simulink model "buses_snt"  (R2025b)
settings: Solver=ode45  StartTime=0.0  StopTime=10.0  RelTol=1e-3  EnableMultiTasking=on
undefined symbols (not defined in the file or in its folder): Rg, Ts
libraries: fl_lib x12, nesl_utility x12, ee_lib x6, eeRmsMeasurement x3
settings Model: Creator=gdudgeon  LastModifiedBy=gdudgeon
settings SolverCC: AlgebraicLoopSolver=TrustRegion
settings DataIOCC: LimitDataPoints=on  SaveFormat=Array  ReturnWorkspaceOutputs=off
settings OptimizationCC: ExpressionDepthLimit=2147483647.0  LifeSpan=inf
settings DebuggingCC: UnderspecifiedInitializationDetection=Classic  MergeDetectMultiDrivingBlocksExec=none  SolverPrmCheckMsg=warning  UnconnectedInputMsg=warning  UnconnectedOutputMsg=warning  UnconnectedLineMsg=warning  StateNameClashWarn=warning  SFUnexpectedBacktrackingDiag=warning  SFNoUnconditionalDefaultTransitionDiag=warning  SFExecutionAtInitializationDiag=none  ArithmeticOperatorsInVariantConditions=warning
settings HardwareCC: ProdBitPerPointer=32.0  ProdBitPerSizeT=32.0  ProdBitPerPtrDiffT=32.0  ProdLargestAtomicFloat=None  ProdIntDivRoundTo=Undefined  ProdEndianess=Unspecified  ProdWordSize=32.0  ProdHWDeviceType=32-bit Generic
settings ModelReferenceCC: EnableRefExpFcnMdlSchedulingChecks=on  PropagateSignalLabelsOutOfModel=off
settings SFSimCC: SimUseLocalCustomCode=off  CustomCodeUndefinedFunction=UseInterfaceOnly
settings RTWCC: RTWUseLocalCustomCode=off  GPUComputeCapability=3.5
settings CodeAppCC: StateflowObjectComments=on
settings GRTTargetCC: TargetLangStandard=C89/C90 (ANSI)
settings ConfigComp: CovMetricSettings=dw  CovSaveCumulativeToWorkspaceVar=on  CovSaveSingleToWorkspaceVar=on  CovExternalEMLEnable=off
settings SimscapeCC: SimscapeNormalizeSystem=off

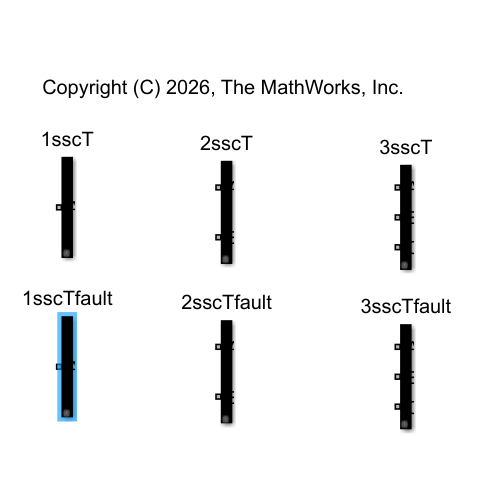
[thumbnail: Simulink's stored preview of the top-level diagram]
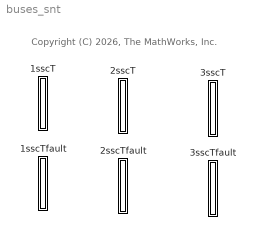
== system buses_snt ==
  note: Copyright (C) 2026, The MathWorks, Inc.
  1sscT : Subsystem  mask{V=4.16e3}
      mask prompts: V "Nominal Voltage (Vrms)"
  1sscTfault : Subsystem  mask{V=4.16e3}
      mask prompts: V "Nominal Voltage (Vrms)"
  2sscT : Subsystem  mask{V=4.16e3}
      mask prompts: V "Nominal Voltage (Vrms)"
  2sscTfault : Subsystem  mask{V=4.16e3}
      mask prompts: V "Nominal Voltage (Vrms)"
  3sscT : Subsystem  mask{V=4.16e3}
      mask prompts: V "Nominal Voltage (Vrms)"
  3sscTfault : Subsystem  mask{V=4.16e3}
      mask prompts: V "Nominal Voltage (Vrms)"

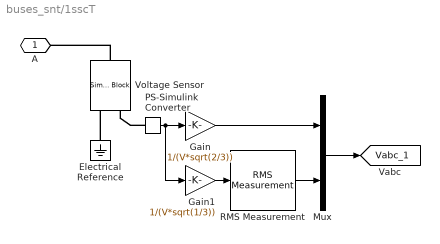
== system buses_snt/1sscT ==
  Electrical Reference : fl_lib/Electrical/Electrical Elements/Electrical Reference
  Gain : Gain  Gain=1/(V*sqrt(2/3))
  Gain1 : Gain  Gain=1/(V*sqrt(1/3))
  Mux : Mux  Inputs=2
  PS-Simulink Converter : nesl_utility/PS-Simulink Converter  PhysicalDomain=network_engine_domain  SubClassName=ps_output  LeftPortType=input  RightPortType=output  PseudoPeriodic=off  Frequencies=[]  VectorFormat=inherit  Unit=inherit  AffineConversion=off
  RMS Measurement : eeRmsMeasurement/RMS Measurement  LabelModeActiveChoice=Total  F=60  SpecifyHarmonics=off  K=[0 1 2]  Ts=Ts
      settings: LibrarySourceBlock=|
      | ee_sl_lib/Measurements/RMS
      | Measurement
  Voltage Sensor : SimscapeComponentBlock  SourceFile=multi_voltage  ComponentPath=multi_voltage  ComponentVariants="[\"multi_voltage\"]"  ComponentVariantNames="[\"multi_voltage\"]"  ClassName=multi_voltage  SchemaVersion=1  noph=1
      settings: CopyFcn=simscape.sscblock.internal.componentBlockCallback(gcbh,'COPY')  PreCopyFcn=simscape.sscblock.internal.componentBlockCallback(gcbh,'PRECOPY')  PreDeleteFcn=simscape.sscblock.internal.componentBlockCallback(gcbh,'PREDELETE')  InternalSimscapePortConfiguration="{\"Bottom\":[],\"Left\":[{\"id\":\"p\",\"label\":\"+\",\"type\":\"foundation.electrical.electrical\"}],\"Right\":[{\"id\":\"V\",\"label\":\"V\",\"type\":\"output\"},{\"id\":\"n\",\"label\":\"-\",\"type\":\"foundation.electrical.electrical\"}],\"Top\":[]}"
      mask Type: Multi-Phase Voltage Sensor
  A : PMIOPort  Side=Left
  tag scope: Vabc_1=global
  wires:
  PS-Simulink Converter/1 -> Gain1/1, Gain/1
  Gain1/1 -> RMS Measurement/1
  RMS Measurement/1 -> Mux/2
  Gain/1 -> Mux/1
  Mux/1 -> [Vabc_1]
  connections:
  PS-Simulink Converter/LConn1 -- Voltage Sensor/RConn1
  Voltage Sensor/LConn1 -- A/RConn1
  Electrical Reference/LConn1 -- Voltage Sensor/RConn2

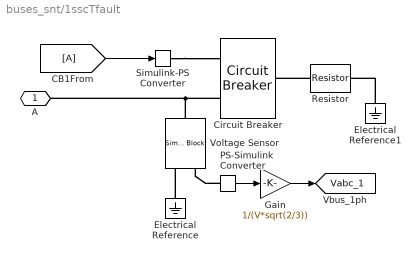
== system buses_snt/1sscTfault ==
  CB1From : From
  Circuit Breaker : ee_lib/Switches & Breakers/Circuit Breaker  R_closed=Ron Ohm  G_open=Goff 1/Ohm  threshold=0.5 V  breaker_behavior=ee.enum.switches.breakerBehavior.zeroCrossingEnable
      settings: InternalSimscapePortConfiguration="{\"Bottom\":[],\"Left\":[{\"id\":\"vT\",\"label\":\"vT\",\"type\":\"input\"},{\"id\":\"p1\",\"label\":\"\",\"type\":\"foundation.electrical.electrical\"}],\"Right\":[{\"id\":\"p2\",\"label\":\"\",\"type\":\"foundation.electrical.electrical\"}],\"Top\":[]}"
  Electrical Reference : fl_lib/Electrical/Electrical Elements/Electrical Reference
  Electrical Reference1 : fl_lib/Electrical/Electrical Elements/Electrical Reference
  Gain : Gain  Gain=1/(V*sqrt(2/3))
  PS-Simulink Converter : nesl_utility/PS-Simulink Converter  PhysicalDomain=network_engine_domain  SubClassName=ps_output  LeftPortType=input  RightPortType=output  PseudoPeriodic=off  Frequencies=[]  VectorFormat=inherit  Unit=inherit  AffineConversion=off
  Resistor : fl_lib/Electrical/Electrical Elements/Resistor  R=Rg Ohm  i_specify=off  i_priority=None  i=0 A  i_nominal_specify=off  i_nominal_value=1  i_nominal_unit=A  v_specify=off  v_priority=None  v=0 V  v_nominal_specify=off  v_nominal_value=1  v_nominal_unit=V
  Simulink-PS Converter : nesl_utility/Simulink-PS Converter  PhysicalDomain=network_engine_domain  SubClassName=ps_input  LeftPortType=input  RightPortType=output  PseudoPeriodic=off  Frequencies=[]  NoiseDistribution=none  NoiseParameters=[]  Unit=1  AffineConversion=off  FilteringAndDerivatives=zero  SimscapeFilterOrder=1  InputFilterTimeConstant=0.001  UdotUserProvided=0
  Voltage Sensor : SimscapeComponentBlock  SourceFile=multi_voltage  ComponentPath=multi_voltage  ComponentVariants="[\"multi_voltage\"]"  ComponentVariantNames="[\"multi_voltage\"]"  ClassName=multi_voltage  SchemaVersion=1  noph=1
      settings: CopyFcn=simscape.sscblock.internal.componentBlockCallback(gcbh,'COPY')  PreCopyFcn=simscape.sscblock.internal.componentBlockCallback(gcbh,'PRECOPY')  PreDeleteFcn=simscape.sscblock.internal.componentBlockCallback(gcbh,'PREDELETE')  InternalSimscapePortConfiguration="{\"Bottom\":[],\"Left\":[{\"id\":\"p\",\"label\":\"+\",\"type\":\"foundation.electrical.electrical\"}],\"Right\":[{\"id\":\"V\",\"label\":\"V\",\"type\":\"output\"},{\"id\":\"n\",\"label\":\"-\",\"type\":\"foundation.electrical.electrical\"}],\"Top\":[]}"
      mask Type: Multi-Phase Voltage Sensor
  A : PMIOPort  Side=Left
  tag scope: Vabc_1=global
  wires:
  Gain/1 -> [Vabc_1]
  PS-Simulink Converter/1 -> Gain/1
  CB1From/1 -> Simulink-PS Converter/1
  connections:
  Electrical Reference/LConn1 -- Voltage Sensor/RConn2
  Voltage Sensor/LConn1 -- A/RConn1 -- Circuit Breaker/LConn2
  PS-Simulink Converter/LConn1 -- Voltage Sensor/RConn1
  Electrical Reference1/LConn1 -- Resistor/RConn1
  Resistor/LConn1 -- Circuit Breaker/RConn1
  Simulink-PS Converter/RConn1 -- Circuit Breaker/LConn1

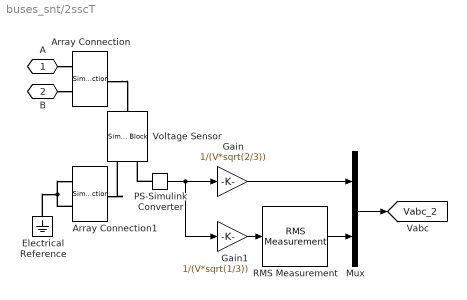
== system buses_snt/2sscT ==
  Array Connection : SimscapeArrayConnection
  Array Connection1 : SimscapeArrayConnection
  Electrical Reference : fl_lib/Electrical/Electrical Elements/Electrical Reference
  Gain : Gain  Gain=1/(V*sqrt(2/3))
  Gain1 : Gain  Gain=1/(V*sqrt(1/3))
  Mux : Mux  Inputs=2
  PS-Simulink Converter : nesl_utility/PS-Simulink Converter  PhysicalDomain=network_engine_domain  SubClassName=ps_output  LeftPortType=input  RightPortType=output  PseudoPeriodic=off  Frequencies=[]  VectorFormat=inherit  Unit=inherit  AffineConversion=off
  RMS Measurement : eeRmsMeasurement/RMS Measurement  LabelModeActiveChoice=Total  F=60  SpecifyHarmonics=off  K=[0 1 2]  Ts=Ts
      settings: LibrarySourceBlock=|
      | ee_sl_lib/Measurements/RMS
      | Measurement
  Voltage Sensor : SimscapeComponentBlock  SourceFile=multi_voltage  ComponentPath=multi_voltage  ComponentVariants="[\"multi_voltage\"]"  ComponentVariantNames="[\"multi_voltage\"]"  ClassName=multi_voltage  SchemaVersion=1  noph=2
      settings: CopyFcn=simscape.sscblock.internal.componentBlockCallback(gcbh,'COPY')  PreCopyFcn=simscape.sscblock.internal.componentBlockCallback(gcbh,'PRECOPY')  PreDeleteFcn=simscape.sscblock.internal.componentBlockCallback(gcbh,'PREDELETE')  InternalSimscapePortConfiguration="{\"Bottom\":[],\"Left\":[{\"id\":\"p\",\"label\":\"+\",\"type\":\"foundation.electrical.electrical\"}],\"Right\":[{\"id\":\"V\",\"label\":\"V\",\"type\":\"output\"},{\"id\":\"n\",\"label\":\"-\",\"type\":\"foundation.electrical.electrical\"}],\"Top\":[]}"
      mask Type: Multi-Phase Voltage Sensor
  A : PMIOPort  Side=Left
  B : PMIOPort  Port=2  Side=Left
  tag scope: Vabc_2=global
  wires:
  Gain1/1 -> RMS Measurement/1
  Mux/1 -> [Vabc_2]
  Gain/1 -> Mux/1
  RMS Measurement/1 -> Mux/2
  PS-Simulink Converter/1 -> Gain1/1, Gain/1
  connections:
  Array Connection/RConn1 -- Voltage Sensor/LConn1
  A/RConn1 -- Array Connection/LConn1
  B/RConn1 -- Array Connection/LConn2
  PS-Simulink Converter/LConn1 -- Voltage Sensor/RConn1
  Array Connection1/RConn1 -- Voltage Sensor/RConn2
  Array Connection1/LConn2 -- Electrical Reference/LConn1 -- Array Connection1/LConn1

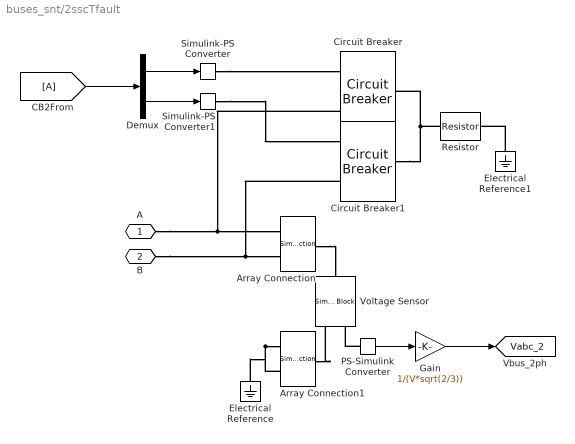
== system buses_snt/2sscTfault ==
  Array Connection : SimscapeArrayConnection
  Array Connection1 : SimscapeArrayConnection
  CB2From : From
  Circuit Breaker : ee_lib/Switches & Breakers/Circuit Breaker  R_closed=Ron Ohm  G_open=Goff 1/Ohm  threshold=0.5 V  breaker_behavior=ee.enum.switches.breakerBehavior.zeroCrossingEnable
      settings: InternalSimscapePortConfiguration="{\"Bottom\":[],\"Left\":[{\"id\":\"vT\",\"label\":\"vT\",\"type\":\"input\"},{\"id\":\"p1\",\"label\":\"\",\"type\":\"foundation.electrical.electrical\"}],\"Right\":[{\"id\":\"p2\",\"label\":\"\",\"type\":\"foundation.electrical.electrical\"}],\"Top\":[]}"
  Circuit Breaker1 : ee_lib/Switches & Breakers/Circuit Breaker  R_closed=Ron Ohm  G_open=Goff 1/Ohm  threshold=0.5 V  breaker_behavior=ee.enum.switches.breakerBehavior.zeroCrossingEnable
      settings: InternalSimscapePortConfiguration="{\"Bottom\":[],\"Left\":[{\"id\":\"vT\",\"label\":\"vT\",\"type\":\"input\"},{\"id\":\"p1\",\"label\":\"\",\"type\":\"foundation.electrical.electrical\"}],\"Right\":[{\"id\":\"p2\",\"label\":\"\",\"type\":\"foundation.electrical.electrical\"}],\"Top\":[]}"
  Demux : Demux  Outputs=2
  Electrical Reference : fl_lib/Electrical/Electrical Elements/Electrical Reference
  Electrical Reference1 : fl_lib/Electrical/Electrical Elements/Electrical Reference
  Gain : Gain  Gain=1/(V*sqrt(2/3))
  PS-Simulink Converter : nesl_utility/PS-Simulink Converter  PhysicalDomain=network_engine_domain  SubClassName=ps_output  LeftPortType=input  RightPortType=output  PseudoPeriodic=off  Frequencies=[]  VectorFormat=inherit  Unit=inherit  AffineConversion=off
  Resistor : fl_lib/Electrical/Electrical Elements/Resistor  R=Rg Ohm  i_specify=off  i_priority=None  i=0 A  i_nominal_specify=off  i_nominal_value=1  i_nominal_unit=A  v_specify=off  v_priority=None  v=0 V  v_nominal_specify=off  v_nominal_value=1  v_nominal_unit=V
  Simulink-PS Converter : nesl_utility/Simulink-PS Converter  PhysicalDomain=network_engine_domain  SubClassName=ps_input  LeftPortType=input  RightPortType=output  PseudoPeriodic=off  Frequencies=[]  NoiseDistribution=none  NoiseParameters=[]  Unit=1  AffineConversion=off  FilteringAndDerivatives=zero  SimscapeFilterOrder=1  InputFilterTimeConstant=0.001  UdotUserProvided=0
  Simulink-PS Converter1 : nesl_utility/Simulink-PS Converter  PhysicalDomain=network_engine_domain  SubClassName=ps_input  LeftPortType=input  RightPortType=output  PseudoPeriodic=off  Frequencies=[]  NoiseDistribution=none  NoiseParameters=[]  Unit=1  AffineConversion=off  FilteringAndDerivatives=zero  SimscapeFilterOrder=1  InputFilterTimeConstant=0.001  UdotUserProvided=0
  Voltage Sensor : SimscapeComponentBlock  SourceFile=multi_voltage  ComponentPath=multi_voltage  ComponentVariants="[\"multi_voltage\"]"  ComponentVariantNames="[\"multi_voltage\"]"  ClassName=multi_voltage  SchemaVersion=1  noph=2
      settings: CopyFcn=simscape.sscblock.internal.componentBlockCallback(gcbh,'COPY')  PreCopyFcn=simscape.sscblock.internal.componentBlockCallback(gcbh,'PRECOPY')  PreDeleteFcn=simscape.sscblock.internal.componentBlockCallback(gcbh,'PREDELETE')  InternalSimscapePortConfiguration="{\"Bottom\":[],\"Left\":[{\"id\":\"p\",\"label\":\"+\",\"type\":\"foundation.electrical.electrical\"}],\"Right\":[{\"id\":\"V\",\"label\":\"V\",\"type\":\"output\"},{\"id\":\"n\",\"label\":\"-\",\"type\":\"foundation.electrical.electrical\"}],\"Top\":[]}"
      mask Type: Multi-Phase Voltage Sensor
  A : PMIOPort  Side=Left
  B : PMIOPort  Port=2  Side=Left
  tag scope: Vabc_2=global
  wires:
  PS-Simulink Converter/1 -> Gain/1
  Gain/1 -> [Vabc_2]
  CB2From/1 -> Demux/1
  Demux/2 -> Simulink-PS Converter1/1
  Demux/1 -> Simulink-PS Converter/1
  connections:
  Array Connection1/LConn1 -- Electrical Reference/LConn1 -- Array Connection1/LConn2
  Array Connection1/RConn1 -- Voltage Sensor/RConn2
  PS-Simulink Converter/LConn1 -- Voltage Sensor/RConn1
  B/RConn1 -- Circuit Breaker1/LConn2 -- Array Connection/LConn2
  A/RConn1 -- Circuit Breaker/LConn2 -- Array Connection/LConn1
  Array Connection/RConn1 -- Voltage Sensor/LConn1
  Resistor/LConn1 -- Circuit Breaker/RConn1 -- Circuit Breaker1/RConn1
  Electrical Reference1/LConn1 -- Resistor/RConn1
  Simulink-PS Converter1/RConn1 -- Circuit Breaker1/LConn1
  Simulink-PS Converter/RConn1 -- Circuit Breaker/LConn1

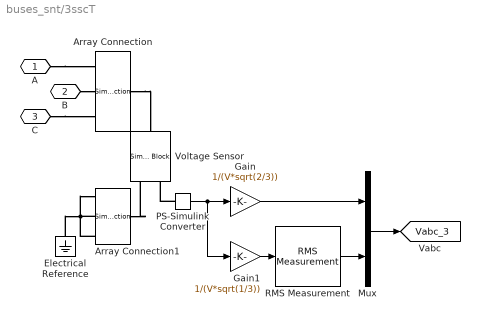
== system buses_snt/3sscT ==
  Array Connection : SimscapeArrayConnection  NumScalarElements=3
  Array Connection1 : SimscapeArrayConnection  NumScalarElements=3
  Electrical Reference : fl_lib/Electrical/Electrical Elements/Electrical Reference
  Gain : Gain  Gain=1/(V*sqrt(2/3))
  Gain1 : Gain  Gain=1/(V*sqrt(1/3))
  Mux : Mux  Inputs=2
  PS-Simulink Converter : nesl_utility/PS-Simulink Converter  PhysicalDomain=network_engine_domain  SubClassName=ps_output  LeftPortType=input  RightPortType=output  PseudoPeriodic=off  Frequencies=[]  VectorFormat=inherit  Unit=inherit  AffineConversion=off
  RMS Measurement : eeRmsMeasurement/RMS Measurement  LabelModeActiveChoice=Total  F=60  SpecifyHarmonics=off  K=[0 1 2]  Ts=Ts
      settings: LibrarySourceBlock=|
      | ee_sl_lib/Measurements/RMS
      | Measurement
  Voltage Sensor : SimscapeComponentBlock  SourceFile=multi_voltage  ComponentPath=multi_voltage  ComponentVariants="[\"multi_voltage\"]"  ComponentVariantNames="[\"multi_voltage\"]"  ClassName=multi_voltage  SchemaVersion=1  noph=3
      settings: CopyFcn=simscape.sscblock.internal.componentBlockCallback(gcbh,'COPY')  PreCopyFcn=simscape.sscblock.internal.componentBlockCallback(gcbh,'PRECOPY')  PreDeleteFcn=simscape.sscblock.internal.componentBlockCallback(gcbh,'PREDELETE')  InternalSimscapePortConfiguration="{\"Bottom\":[],\"Left\":[{\"id\":\"p\",\"label\":\"+\",\"type\":\"foundation.electrical.electrical\"}],\"Right\":[{\"id\":\"V\",\"label\":\"V\",\"type\":\"output\"},{\"id\":\"n\",\"label\":\"-\",\"type\":\"foundation.electrical.electrical\"}],\"Top\":[]}"
      mask Type: Multi-Phase Voltage Sensor
  A : PMIOPort  Side=Left
  B : PMIOPort  Port=2  Side=Left
  C : PMIOPort  Port=3  Side=Left
  tag scope: Vabc_3=global
  wires:
  Gain1/1 -> RMS Measurement/1
  Mux/1 -> [Vabc_3]
  Gain/1 -> Mux/1
  RMS Measurement/1 -> Mux/2
  PS-Simulink Converter/1 -> Gain1/1, Gain/1
  connections:
  Array Connection1/LConn2 -- Array Connection1/LConn1 -- Electrical Reference/LConn1 -- Array Connection1/LConn3
  Array Connection/RConn1 -- Voltage Sensor/LConn1
  PS-Simulink Converter/LConn1 -- Voltage Sensor/RConn1
  Array Connection1/RConn1 -- Voltage Sensor/RConn2
  B/RConn1 -- Array Connection/LConn2
  A/RConn1 -- Array Connection/LConn1
  C/RConn1 -- Array Connection/LConn3

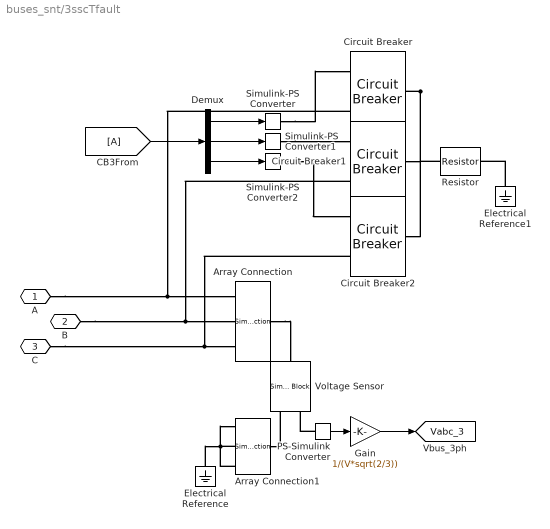
== system buses_snt/3sscTfault ==
  Array Connection : SimscapeArrayConnection  NumScalarElements=3
  Array Connection1 : SimscapeArrayConnection  NumScalarElements=3
  CB3From : From
  Circuit Breaker : ee_lib/Switches & Breakers/Circuit Breaker  R_closed=Ron Ohm  G_open=Goff 1/Ohm  threshold=0.5 V  breaker_behavior=ee.enum.switches.breakerBehavior.zeroCrossingEnable
      settings: InternalSimscapePortConfiguration="{\"Bottom\":[],\"Left\":[{\"id\":\"vT\",\"label\":\"vT\",\"type\":\"input\"},{\"id\":\"p1\",\"label\":\"\",\"type\":\"foundation.electrical.electrical\"}],\"Right\":[{\"id\":\"p2\",\"label\":\"\",\"type\":\"foundation.electrical.electrical\"}],\"Top\":[]}"
  Circuit Breaker1 : ee_lib/Switches & Breakers/Circuit Breaker  R_closed=Ron Ohm  G_open=Goff 1/Ohm  threshold=0.5 V  breaker_behavior=ee.enum.switches.breakerBehavior.zeroCrossingEnable
      settings: InternalSimscapePortConfiguration="{\"Bottom\":[],\"Left\":[{\"id\":\"vT\",\"label\":\"vT\",\"type\":\"input\"},{\"id\":\"p1\",\"label\":\"\",\"type\":\"foundation.electrical.electrical\"}],\"Right\":[{\"id\":\"p2\",\"label\":\"\",\"type\":\"foundation.electrical.electrical\"}],\"Top\":[]}"
  Circuit Breaker2 : ee_lib/Switches & Breakers/Circuit Breaker  R_closed=Ron Ohm  G_open=Goff 1/Ohm  threshold=0.5 V  breaker_behavior=ee.enum.switches.breakerBehavior.zeroCrossingEnable
      settings: InternalSimscapePortConfiguration="{\"Bottom\":[],\"Left\":[{\"id\":\"vT\",\"label\":\"vT\",\"type\":\"input\"},{\"id\":\"p1\",\"label\":\"\",\"type\":\"foundation.electrical.electrical\"}],\"Right\":[{\"id\":\"p2\",\"label\":\"\",\"type\":\"foundation.electrical.electrical\"}],\"Top\":[]}"
  Demux : Demux  Outputs=3
  Electrical Reference : fl_lib/Electrical/Electrical Elements/Electrical Reference
  Electrical Reference1 : fl_lib/Electrical/Electrical Elements/Electrical Reference
  Gain : Gain  Gain=1/(V*sqrt(2/3))
  PS-Simulink Converter : nesl_utility/PS-Simulink Converter  PhysicalDomain=network_engine_domain  SubClassName=ps_output  LeftPortType=input  RightPortType=output  PseudoPeriodic=off  Frequencies=[]  VectorFormat=inherit  Unit=inherit  AffineConversion=off
  Resistor : fl_lib/Electrical/Electrical Elements/Resistor  R=Rg Ohm  i_specify=off  i_priority=None  i=0 A  i_nominal_specify=off  i_nominal_value=1  i_nominal_unit=A  v_specify=off  v_priority=None  v=0 V  v_nominal_specify=off  v_nominal_value=1  v_nominal_unit=V
  Simulink-PS Converter : nesl_utility/Simulink-PS Converter  PhysicalDomain=network_engine_domain  SubClassName=ps_input  LeftPortType=input  RightPortType=output  PseudoPeriodic=off  Frequencies=[]  NoiseDistribution=none  NoiseParameters=[]  Unit=1  AffineConversion=off  FilteringAndDerivatives=zero  SimscapeFilterOrder=1  InputFilterTimeConstant=0.001  UdotUserProvided=0
  Simulink-PS Converter1 : nesl_utility/Simulink-PS Converter  PhysicalDomain=network_engine_domain  SubClassName=ps_input  LeftPortType=input  RightPortType=output  PseudoPeriodic=off  Frequencies=[]  NoiseDistribution=none  NoiseParameters=[]  Unit=1  AffineConversion=off  FilteringAndDerivatives=zero  SimscapeFilterOrder=1  InputFilterTimeConstant=0.001  UdotUserProvided=0
  Simulink-PS Converter2 : nesl_utility/Simulink-PS Converter  PhysicalDomain=network_engine_domain  SubClassName=ps_input  LeftPortType=input  RightPortType=output  PseudoPeriodic=off  Frequencies=[]  NoiseDistribution=none  NoiseParameters=[]  Unit=1  AffineConversion=off  FilteringAndDerivatives=zero  SimscapeFilterOrder=1  InputFilterTimeConstant=0.001  UdotUserProvided=0
  Voltage Sensor : SimscapeComponentBlock  SourceFile=multi_voltage  ComponentPath=multi_voltage  ComponentVariants="[\"multi_voltage\"]"  ComponentVariantNames="[\"multi_voltage\"]"  ClassName=multi_voltage  SchemaVersion=1  noph=3
      settings: CopyFcn=simscape.sscblock.internal.componentBlockCallback(gcbh,'COPY')  PreCopyFcn=simscape.sscblock.internal.componentBlockCallback(gcbh,'PRECOPY')  PreDeleteFcn=simscape.sscblock.internal.componentBlockCallback(gcbh,'PREDELETE')  InternalSimscapePortConfiguration="{\"Bottom\":[],\"Left\":[{\"id\":\"p\",\"label\":\"+\",\"type\":\"foundation.electrical.electrical\"}],\"Right\":[{\"id\":\"V\",\"label\":\"V\",\"type\":\"output\"},{\"id\":\"n\",\"label\":\"-\",\"type\":\"foundation.electrical.electrical\"}],\"Top\":[]}"
      mask Type: Multi-Phase Voltage Sensor
  A : PMIOPort  Side=Left
  B : PMIOPort  Port=2  Side=Left
  C : PMIOPort  Port=3  Side=Left
  tag scope: Vabc_3=global
  wires:
  PS-Simulink Converter/1 -> Gain/1
  Gain/1 -> [Vabc_3]
  CB3From/1 -> Demux/1
  Demux/2 -> Simulink-PS Converter1/1
  Demux/1 -> Simulink-PS Converter/1
  Demux/3 -> Simulink-PS Converter2/1
  connections:
  C/RConn1 -- Circuit Breaker2/LConn2 -- Array Connection/LConn3
  A/RConn1 -- Circuit Breaker/LConn2 -- Array Connection/LConn1
  B/RConn1 -- Circuit Breaker1/LConn2 -- Array Connection/LConn2
  Array Connection1/RConn1 -- Voltage Sensor/RConn2
  PS-Simulink Converter/LConn1 -- Voltage Sensor/RConn1
  Array Connection/RConn1 -- Voltage Sensor/LConn1
  Array Connection1/LConn3 -- Electrical Reference/LConn1 -- Array Connection1/LConn1 -- Array Connection1/LConn2
  Circuit Breaker/RConn1 -- Circuit Breaker2/RConn1 -- Resistor/LConn1 -- Circuit Breaker1/RConn1
  Simulink-PS Converter1/RConn1 -- Circuit Breaker1/LConn1
  Simulink-PS Converter/RConn1 -- Circuit Breaker/LConn1
  Simulink-PS Converter2/RConn1 -- Circuit Breaker2/LConn1
  Electrical Reference1/LConn1 -- Resistor/RConn1
